simulink library "xbsDSP48_r3"  (Simulink 5.0)
libraries: xbsIndex_r3 x429, xbsDSP48_r3 x2
(part 4 of 8)

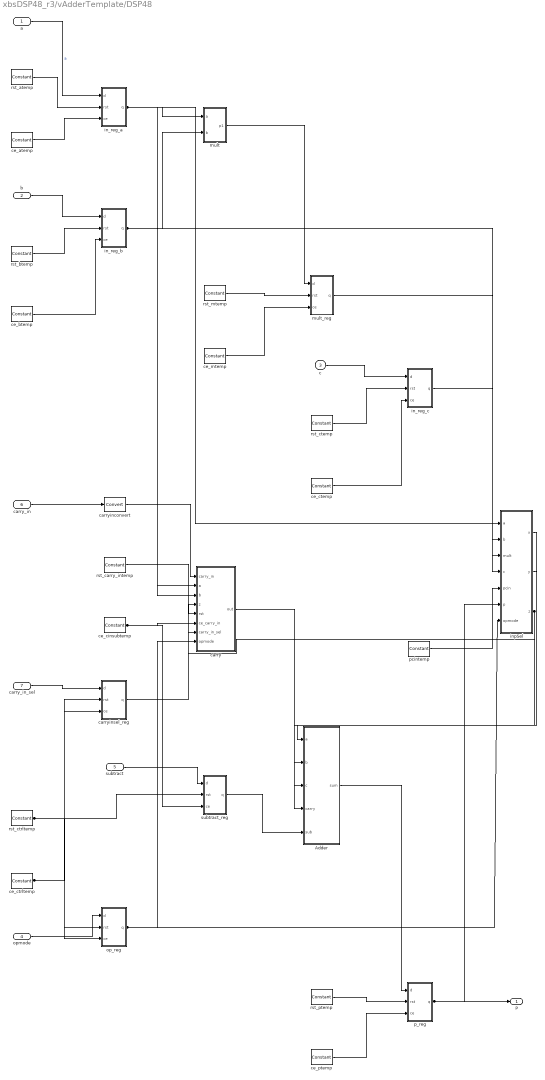
== system xbsDSP48_r3/vAdderTemplate/DSP48 ==
  a : Inport
  b : Inport  Port=2
  c : Inport  Port=3
  opmode : Inport  Port=4
  subtract : Inport  Port=5
  carry_in : Inport  Port=6
  carry_in_sel : Inport  Port=7
  Adder : Subsystem
  carry : Subsystem
  carryinconvert : xbsIndex_r3/Convert  arith_type=Unsigned  n_bits=1  bin_pt=0  quantization=Truncate  overflow=Wrap  latency=0  explicit_period=off  period=1  dbl_ovrd=off  show_param=off  inserted_by_tool=off  pipeline=off
      settings: xl_area=[0, 0, 0, 0, 0, 0, 0]
  carryinsel_reg : Subsystem  mask{nreg=pipeline_carryinsel, pnreg=1}
      mask prompts: nreg "Number of registers"; pnreg "Previous number of register"
      mask init: same as xbsDSP48_r3/DSP48reg
      mask Display:
      | patch([0 iWidth iWidth 0],[0 0 iHeight iHeight] , bg);
      | patch(logoX,logoY , fg);
      | text(iCx-6,iCy,'z');
      | text(iCx,iCy+4,str);
      | port_label('input',1,'d');
      | port_label('input',2,'rst');
      | port_label('input',3,'ce');
      | port_label('output',1,'q');
      | plot([0 0 iWidth iWidth 0], [0 iHeight iHeight 0 0]);
  ce_atemp : xbsIndex_r3/Constant  const=1  equ=P=C  arith_type=Boolean  n_bits=1  bin_pt=0  opselect=C  inp2=PCIN>>17  opr=+  inp1=P  carry=CIN  iostate=0  explicit_period=on  period=2  dbl_ovrd=off
  ce_btemp : xbsIndex_r3/Constant  const=1  equ=P=C  arith_type=Boolean  n_bits=1  bin_pt=0  opselect=C  inp2=PCIN>>17  opr=+  inp1=P  carry=CIN  iostate=0  explicit_period=on  period=2  dbl_ovrd=off
  ce_cinsubtemp : xbsIndex_r3/Constant  const=1  equ=P=C  arith_type=Boolean  n_bits=1  bin_pt=0  opselect=C  inp2=PCIN>>17  opr=+  inp1=P  carry=CIN  iostate=0  explicit_period=on  period=2  dbl_ovrd=off
  ce_ctemp : xbsIndex_r3/Constant  const=1  equ=P=C  arith_type=Boolean  n_bits=1  bin_pt=0  opselect=C  inp2=PCIN>>17  opr=+  inp1=P  carry=CIN  iostate=0  explicit_period=on  period=2  dbl_ovrd=off
  ce_ctrltemp : xbsIndex_r3/Constant  const=1  arith_type=Boolean  n_bits=1  bin_pt=0  explicit_period=on  period=2  dbl_ovrd=off
  ce_mtemp : xbsIndex_r3/Constant  const=1  equ=P=C  arith_type=Boolean  n_bits=1  bin_pt=0  opselect=C  inp2=PCIN>>17  opr=+  inp1=P  carry=CIN  iostate=0  explicit_period=on  period=2  dbl_ovrd=off
  ce_ptemp : xbsIndex_r3/Constant  const=1  arith_type=Boolean  n_bits=1  bin_pt=0  explicit_period=on  period=2  dbl_ovrd=off
  in_reg_a : Subsystem  mask{nreg=pipeline_a-1, pnreg=1}
      mask prompts: nreg "Number of registers"; pnreg "Previous number of register"
      mask init: same as xbsDSP48_r3/DSP48reg
      mask Display:
      | patch([0 iWidth iWidth 0],[0 0 iHeight iHeight] , bg);
      | patch(logoX,logoY , fg);
      | text(iCx-6,iCy,'z');
      | text(iCx,iCy+4,str);
      | port_label('input',1,'d');
      | port_label('input',2,'rst');
      | port_label('input',3,'ce');
      | port_label('output',1,'q');
      | plot([0 0 iWidth iWidth 0], [0 iHeight iHeight 0 0]);
  in_reg_b : Subsystem  mask{nreg=pipeline_b- 1, pnreg=1}
      mask prompts: nreg "Number of registers"; pnreg "Previous number of register"
      mask init: same as xbsDSP48_r3/DSP48reg
      mask Display:
      | patch([0 iWidth iWidth 0],[0 0 iHeight iHeight] , bg);
      | patch(logoX,logoY , fg);
      | text(iCx-6,iCy,'z');
      | text(iCx,iCy+4,str);
      | port_label('input',1,'d');
      | port_label('input',2,'rst');
      | port_label('input',3,'ce');
      | port_label('output',1,'q');
      | plot([0 0 iWidth iWidth 0], [0 iHeight iHeight 0 0]);
  in_reg_c : Subsystem  mask{nreg=pipeline_c, pnreg=1}
      mask prompts: nreg "Number of registers"; pnreg "Previous number of register"
      mask init: same as xbsDSP48_r3/DSP48reg
      mask Display:
      | patch([0 iWidth iWidth 0],[0 0 iHeight iHeight] , bg);
      | patch(logoX,logoY , fg);
      | text(iCx-6,iCy,'z');
      | text(iCx,iCy+4,str);
      | port_label('input',1,'d');
      | port_label('input',2,'rst');
      | port_label('input',3,'ce');
      | port_label('output',1,'q');
      | plot([0 0 iWidth iWidth 0], [0 iHeight iHeight 0 0]);
  inpSel : Subsystem
  mult : Subsystem
  mult_reg : Subsystem  mask{nreg=pipeline_mult, pnreg=1}
      mask prompts: nreg "Number of registers"; pnreg "Previous number of register"
      mask init: same as xbsDSP48_r3/DSP48reg
      mask Display:
      | patch([0 iWidth iWidth 0],[0 0 iHeight iHeight] , bg);
      | patch(logoX,logoY , fg);
      | text(iCx-6,iCy,'z');
      | text(iCx,iCy+4,str);
      | port_label('input',1,'d');
      | port_label('input',2,'rst');
      | port_label('input',3,'ce');
      | port_label('output',1,'q');
      | plot([0 0 iWidth iWidth 0], [0 iHeight iHeight 0 0]);
  op_reg : Subsystem  mask{nreg=pipeline_opmode, pnreg=1}
      mask prompts: nreg "Number of registers"; pnreg "Previous number of register"
      mask init: same as xbsDSP48_r3/DSP48reg
      mask Display:
      | patch([0 iWidth iWidth 0],[0 0 iHeight iHeight] , bg);
      | patch(logoX,logoY , fg);
      | text(iCx-6,iCy,'z');
      | text(iCx,iCy+4,str);
      | port_label('input',1,'d');
      | port_label('input',2,'rst');
      | port_label('input',3,'ce');
      | port_label('output',1,'q');
      | plot([0 0 iWidth iWidth 0], [0 iHeight iHeight 0 0]);
  p_reg : Subsystem  mask{nreg=pipeline_p, pnreg=1}
      mask prompts: nreg "Number of registers"; pnreg "Previous number of register"
      mask init: same as xbsDSP48_r3/DSP48reg
      mask Display:
      | patch([0 iWidth iWidth 0],[0 0 iHeight iHeight] , bg);
      | patch(logoX,logoY , fg);
      | text(iCx-6,iCy,'z');
      | text(iCx,iCy+4,str);
      | port_label('input',1,'d');
      | port_label('input',2,'rst');
      | port_label('input',3,'ce');
      | port_label('output',1,'q');
      | plot([0 0 iWidth iWidth 0], [0 iHeight iHeight 0 0]);
  pcintemp : xbsIndex_r3/Constant  const=1  equ=P=C  arith_type="Signed  (2's comp)"  n_bits=48  bin_pt=0  opselect=C  inp2=PCIN>>17  opr=+  inp1=P  carry=CIN  iostate=0  explicit_period=on  period=2  dbl_ovrd=off
  rst_atemp : xbsIndex_r3/Constant  const=0  equ=P=C  arith_type=Boolean  n_bits=1  bin_pt=0  opselect=C  inp2=PCIN>>17  opr=+  inp1=P  carry=CIN  iostate=0  explicit_period=on  period=2  dbl_ovrd=off
  rst_btemp : xbsIndex_r3/Constant  const=0  equ=P=C  arith_type=Boolean  n_bits=1  bin_pt=0  opselect=C  inp2=PCIN>>17  opr=+  inp1=P  carry=CIN  iostate=0  explicit_period=on  period=2  dbl_ovrd=off
  rst_carry_intemp : xbsIndex_r3/Constant  const=0  equ=P=C  arith_type=Boolean  n_bits=1  bin_pt=0  opselect=C  inp2=PCIN>>17  opr=+  inp1=P  carry=CIN  iostate=0  explicit_period=on  period=2  dbl_ovrd=off
  rst_ctemp : xbsIndex_r3/Constant  const=0  equ=P=C  arith_type=Boolean  n_bits=1  bin_pt=0  opselect=C  inp2=PCIN>>17  opr=+  inp1=P  carry=CIN  iostate=0  explicit_period=on  period=2  dbl_ovrd=off
  rst_ctrltemp : xbsIndex_r3/Constant  const=0  equ=P=C  arith_type=Boolean  n_bits=1  bin_pt=0  opselect=C  inp2=PCIN>>17  opr=+  inp1=P  carry=CIN  iostate=0  explicit_period=on  period=2  dbl_ovrd=off
  rst_mtemp : xbsIndex_r3/Constant  const=0  equ=P=C  arith_type=Boolean  n_bits=1  bin_pt=0  opselect=C  inp2=PCIN>>17  opr=+  inp1=P  carry=CIN  iostate=0  explicit_period=on  period=2  dbl_ovrd=off
  rst_ptemp : xbsIndex_r3/Constant  const=0  arith_type=Boolean  n_bits=1  bin_pt=0  explicit_period=on  period=2  dbl_ovrd=off
  subtract_reg : Subsystem  mask{nreg=pipeline_sub, pnreg=1}
      mask prompts: nreg "Number of registers"; pnreg "Previous number of register"
      mask init: same as xbsDSP48_r3/DSP48reg
      mask Display:
      | patch([0 iWidth iWidth 0],[0 0 iHeight iHeight] , bg);
      | patch(logoX,logoY , fg);
      | text(iCx-6,iCy,'z');
      | text(iCx,iCy+4,str);
      | port_label('input',1,'d');
      | port_label('input',2,'rst');
      | port_label('input',3,'ce');
      | port_label('output',1,'q');
      | plot([0 0 iWidth iWidth 0], [0 iHeight iHeight 0 0]);
  P : Outport
  wires:
  ce_cinsubtemp/1 -> carry/6(ce_carry_in), subtract_reg/3(ce)
  ce_ctrltemp/1 -> carryinsel_reg/3(ce), op_reg/3(ce)
  rst_ctrltemp/1 -> op_reg/2(rst), subtract_reg/2(rst), carryinsel_reg/2(rst)
  p_reg/1(q) -> P/1, inpSel/6(p)
  in_reg_b/1(q) -> mult/2(b), inpSel/2(b), carry/3(b)
  op_reg/1(q) -> inpSel/7(opmode), carry/8(opmode)
  inpSel/3(z) -> Adder/3(c), carry/4(z)
  in_reg_a/1(q) -> mult/1(a), carry/2(a), inpSel/1(a)
  c/1 -> in_reg_c/1(d)
  carryinconvert/1 -> carry/1(carry_in)
  in_reg_c/1(q) -> inpSel/4(c)
  mult/1(p1) -> mult_reg/1(d)
  mult_reg/1(q) -> inpSel/3(mult)
  inpSel/1(x) -> Adder/1(a)
  inpSel/2(y) -> Adder/2(b)
  Adder/1(sum) -> p_reg/1(d)
  subtract_reg/1(q) -> Adder/5(sub)
  carry/1(out) -> Adder/4(carry)
  subtract/1 -> subtract_reg/1(d)
  a/1 -> in_reg_a/1(d)  "a"
  opmode/1 -> op_reg/1(d)
  carry_in/1 -> carryinconvert/1
  carry_in_sel/1 -> carryinsel_reg/1(d)
  carryinsel_reg/1(q) -> carry/7(carry_in_sel)
  b/1 -> in_reg_b/1(d)
  rst_atemp/1 -> in_reg_a/2(rst)
  rst_btemp/1 -> in_reg_b/2(rst)
  rst_ctemp/1 -> in_reg_c/2(rst)
  rst_ptemp/1 -> p_reg/2(rst)
  rst_mtemp/1 -> mult_reg/2(rst)
  rst_carry_intemp/1 -> carry/5(rst)
  ce_atemp/1 -> in_reg_a/3(ce)
  ce_btemp/1 -> in_reg_b/3(ce)
  ce_ctemp/1 -> in_reg_c/3(ce)
  ce_ptemp/1 -> p_reg/3(ce)
  ce_mtemp/1 -> mult_reg/3(ce)
  pcintemp/1 -> inpSel/5(pcin)
